simulink model "carro"  (Simulink 8.7)
settings: Solver=ode3  StartTime=0.0  StopTime=8  FixedStep=0.001  RelTol=1e-3
settings Model: Creator=Dinis  LastModifiedBy=Dinis
settings DataIOCC: LimitDataPoints=off  SaveFormat=Dataset
settings DebuggingCC: UnderspecifiedInitializationDetection=Simplified  MergeDetectMultiDrivingBlocksExec=error
settings HardwareCC: ProdBitPerPointer=64  ProdLargestAtomicFloat=Float  ProdIntDivRoundTo=Zero  ProdEndianess=LittleEndian  ProdHWDeviceType=Specified
settings ModelReferenceCC: PropagateSignalLabelsOutOfModel=on
settings ConfigComp: CovModelRefEnable=off

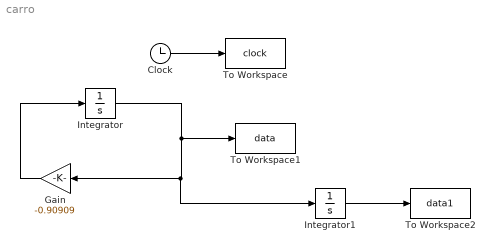
== system carro ==
  Clock : Clock
  Gain : Gain  Gain=-0.90909
  Integrator : Integrator  InitialCondition=-3
  Integrator1 : Integrator  InitialCondition=5
  To Workspace : ToWorkspace  VariableName=clock  SampleTime=-1
  To Workspace1 : ToWorkspace  VariableName=data  SampleTime=-1
  To Workspace2 : ToWorkspace  VariableName=data1  SampleTime=-1
  wires:
  Gain/1 -> Integrator/1
  Clock/1 -> To Workspace/1
  Integrator/1 -> Integrator1/1, Gain/1, To Workspace1/1
  Integrator1/1 -> To Workspace2/1
